simulink model "euler321_I2B_12B_with_contracts_ALL"  (R2019b)
settings: Solver=ode3  StartTime=0.0  StopTime=10.0  FixedStep=0.01  RelTol=1e-3  EnableMultiTasking=on
model workspace (MAT data in the model file):
  ContractValidatorBlocksMap : containers.Map (value not decoded)
undefined symbols (not defined in the file): contractAfterSimulation, contractBeforeSimulation, ContractBlock, ContractGuaranteeBlock, ContractValidatorBlock, saveValidatorParameters
libraries: cocosimLibs x1
(part 2 of 2)

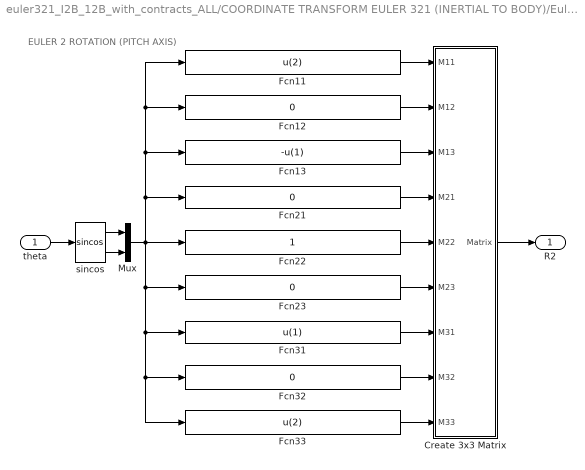
== system euler321_I2B_12B_with_contracts_ALL/COORDINATE TRANSFORM EULER 321 (INERTIAL TO BODY)/Euler 2 Rotation (Pitch) ==
  note: EULER 2 ROTATION (PITCH AXIS)
  theta : Inport
  Create 3x3 Matrix : Subsystem  mask(Create 3x3 Matrix){}
      mask help: shared_aeroblks:sharedaeroblkutil:blockCreate3x3MatrixDesc
      mask init:
      | if license('test','aerospace_blockset')
      |     aerosharedicon('shared');
      | elseif license('test','powertrain_blockset')
      |     sharedautoicon('shared');
      | end
      mask Help: eval('if license(''test'',''aerospace_blockset'')aerosharedhelp(''create_threebythree_matrix'');elseif license(''test'',''powertrain_blockset'')sharedautohelp(''create_threebythree_matrix'');end')
      mask Display:
      | port_label('input',1,'A_{11}','texmode','on');
      | port_label('input',2,'A_{12}','texmode','on');
      | port_label('input',3,'A_{13}','texmode','on');
      | port_label('input',4,'A_{21}','texmode','on');
      | port_label('input',5,'A_{22}','texmode','on');
      | port_label('input',6,'A_{23}','texmode','on');
      | port_label('input',7,'A_{31}','texmode','on');
      | port_label('input',8,'A_{32}','texmode','on');
      | port_label('input',9,'A_{33}','texmode','on');
      | port_label('output',1,'A','texmode','on');
  Fcn11 : Fcn  Expr=u(2)
  Fcn{12,21,23,32} (4 alike) : Fcn  Expr=0
  Fcn13 : Fcn  Expr=-u(1)
  Fcn22 : Fcn  Expr=1
  Fcn31 : Fcn  Expr=u(1)
  Fcn33 : Fcn  Expr=u(2)
  Mux : Mux  Inputs=2
  sincos : Trigonometry  Operator=sincos
  R2 : Outport  PortDimensions=[3,3]  VectorParamsAs1DForOutWhenUnconnected=off
  wires:
  theta/1 -> sincos/1
  Create 3x3 Matrix/1(Matrix) -> R2/1
  sincos/1 -> Mux/1
  sincos/2 -> Mux/2
  Mux/1 -> Fcn32/1, Fcn33/1, Fcn31/1, Fcn23/1, Fcn22/1, Fcn11/1, Fcn12/1, Fcn13/1, Fcn21/1
  Fcn11/1 -> Create 3x3 Matrix/1(M11)
  Fcn12/1 -> Create 3x3 Matrix/2(M12)
  Fcn13/1 -> Create 3x3 Matrix/3(M13)
  Fcn21/1 -> Create 3x3 Matrix/4(M21)
  Fcn31/1 -> Create 3x3 Matrix/7(M31)
  Fcn22/1 -> Create 3x3 Matrix/5(M22)
  Fcn23/1 -> Create 3x3 Matrix/6(M23)
  Fcn32/1 -> Create 3x3 Matrix/8(M32)
  Fcn33/1 -> Create 3x3 Matrix/9(M33)

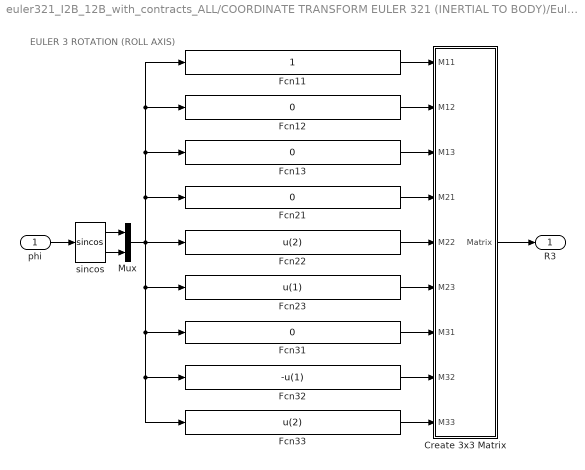
== system euler321_I2B_12B_with_contracts_ALL/COORDINATE TRANSFORM EULER 321 (INERTIAL TO BODY)/Euler 3 Rotation (Roll) ==
  note: EULER 3 ROTATION (ROLL AXIS)
  phi : Inport
  Create 3x3 Matrix : Subsystem  mask(Create 3x3 Matrix){}
      mask help: shared_aeroblks:sharedaeroblkutil:blockCreate3x3MatrixDesc
      mask init:
      | if license('test','aerospace_blockset')
      |     aerosharedicon('shared');
      | elseif license('test','powertrain_blockset')
      |     sharedautoicon('shared');
      | end
      mask Help: eval('if license(''test'',''aerospace_blockset'')aerosharedhelp(''create_threebythree_matrix'');elseif license(''test'',''powertrain_blockset'')sharedautohelp(''create_threebythree_matrix'');end')
      mask Display:
      | port_label('input',1,'A_{11}','texmode','on');
      | port_label('input',2,'A_{12}','texmode','on');
      | port_label('input',3,'A_{13}','texmode','on');
      | port_label('input',4,'A_{21}','texmode','on');
      | port_label('input',5,'A_{22}','texmode','on');
      | port_label('input',6,'A_{23}','texmode','on');
      | port_label('input',7,'A_{31}','texmode','on');
      | port_label('input',8,'A_{32}','texmode','on');
      | port_label('input',9,'A_{33}','texmode','on');
      | port_label('output',1,'A','texmode','on');
  Fcn11 : Fcn  Expr=1
  Fcn{12..13,21,31} (4 alike) : Fcn  Expr=0
  Fcn22 : Fcn  Expr=u(2)
  Fcn23 : Fcn  Expr=u(1)
  Fcn32 : Fcn  Expr=-u(1)
  Fcn33 : Fcn  Expr=u(2)
  Mux : Mux  Inputs=2
  sincos : Trigonometry  Operator=sincos
  R3 : Outport  PortDimensions=[3,3]  VectorParamsAs1DForOutWhenUnconnected=off
  wires:
  phi/1 -> sincos/1
  Create 3x3 Matrix/1(Matrix) -> R3/1
  sincos/1 -> Mux/1
  sincos/2 -> Mux/2
  Mux/1 -> Fcn32/1, Fcn33/1, Fcn31/1, Fcn23/1, Fcn22/1, Fcn11/1, Fcn12/1, Fcn13/1, Fcn21/1
  Fcn11/1 -> Create 3x3 Matrix/1(M11)
  Fcn12/1 -> Create 3x3 Matrix/2(M12)
  Fcn13/1 -> Create 3x3 Matrix/3(M13)
  Fcn21/1 -> Create 3x3 Matrix/4(M21)
  Fcn31/1 -> Create 3x3 Matrix/7(M31)
  Fcn22/1 -> Create 3x3 Matrix/5(M22)
  Fcn23/1 -> Create 3x3 Matrix/6(M23)
  Fcn32/1 -> Create 3x3 Matrix/8(M32)
  Fcn33/1 -> Create 3x3 Matrix/9(M33)

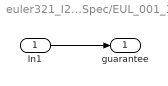
== system euler321_I2B_12B_with_contracts_ALL/euler321_I2B_12B_euler321_Spec/EUL_001_1 ==
  In1 : Inport
  guarantee : Outport  OutDataTypeStr=boolean
  wires:
  In1/1 -> guarantee/1

== system euler321_I2B_12B_with_contracts_ALL/euler321_I2B_12B_euler321_Spec/EUL_001_2 ==
  In1 : Inport
  guarantee : Outport  OutDataTypeStr=boolean
  wires:
  In1/1 -> guarantee/1

== system euler321_I2B_12B_with_contracts_ALL/euler321_I2B_12B_euler321_Spec/EUL_001_3 ==
  In1 : Inport
  guarantee : Outport  OutDataTypeStr=boolean
  wires:
  In1/1 -> guarantee/1

== system euler321_I2B_12B_with_contracts_ALL/euler321_I2B_12B_euler321_Spec/EUL_001_4 ==
  In1 : Inport
  guarantee : Outport  OutDataTypeStr=boolean
  wires:
  In1/1 -> guarantee/1

== system euler321_I2B_12B_with_contracts_ALL/euler321_I2B_12B_euler321_Spec/EUL_001_5 ==
  In1 : Inport
  guarantee : Outport  OutDataTypeStr=boolean
  wires:
  In1/1 -> guarantee/1

== system euler321_I2B_12B_with_contracts_ALL/euler321_I2B_12B_euler321_Spec/EUL_001_6 ==
  In1 : Inport
  guarantee : Outport  OutDataTypeStr=boolean
  wires:
  In1/1 -> guarantee/1

== system euler321_I2B_12B_with_contracts_ALL/euler321_I2B_12B_euler321_Spec/EUL_001_7 ==
  In1 : Inport
  guarantee : Outport  OutDataTypeStr=boolean
  wires:
  In1/1 -> guarantee/1

== system euler321_I2B_12B_with_contracts_ALL/euler321_I2B_12B_euler321_Spec/EUL_001_8 ==
  In1 : Inport
  guarantee : Outport  OutDataTypeStr=boolean
  wires:
  In1/1 -> guarantee/1

== system euler321_I2B_12B_with_contracts_ALL/euler321_I2B_12B_euler321_Spec/EUL_001_9 ==
  In1 : Inport
  guarantee : Outport  OutDataTypeStr=boolean
  wires:
  In1/1 -> guarantee/1

== system euler321_I2B_12B_with_contracts_ALL/euler321_I2B_12B_euler321_Spec/EUL_002_1 ==
  In1 : Inport
  guarantee : Outport  OutDataTypeStr=boolean
  wires:
  In1/1 -> guarantee/1

== system euler321_I2B_12B_with_contracts_ALL/euler321_I2B_12B_euler321_Spec/EUL_002_2 ==
  In1 : Inport
  guarantee : Outport  OutDataTypeStr=boolean
  wires:
  In1/1 -> guarantee/1

== system euler321_I2B_12B_with_contracts_ALL/euler321_I2B_12B_euler321_Spec/EUL_002_3 ==
  In1 : Inport
  guarantee : Outport  OutDataTypeStr=boolean
  wires:
  In1/1 -> guarantee/1

== system euler321_I2B_12B_with_contracts_ALL/euler321_I2B_12B_euler321_Spec/EUL_003 ==
  In1 : Inport
  guarantee : Outport  OutDataTypeStr=boolean
  wires:
  In1/1 -> guarantee/1

== system euler321_I2B_12B_with_contracts_ALL/euler321_I2B_12B_euler321_Spec/EUL_004 ==
  In1 : Inport
  guarantee : Outport  OutDataTypeStr=boolean
  wires:
  In1/1 -> guarantee/1

== system euler321_I2B_12B_with_contracts_ALL/euler321_I2B_12B_euler321_Spec/EUL_006_1 ==
  In1 : Inport
  guarantee : Outport  OutDataTypeStr=boolean
  wires:
  In1/1 -> guarantee/1

== system euler321_I2B_12B_with_contracts_ALL/euler321_I2B_12B_euler321_Spec/EUL_006_2 ==
  In1 : Inport
  guarantee : Outport  OutDataTypeStr=boolean
  wires:
  In1/1 -> guarantee/1

== system euler321_I2B_12B_with_contracts_ALL/euler321_I2B_12B_euler321_Spec/EUL_006_3 ==
  In1 : Inport
  guarantee : Outport  OutDataTypeStr=boolean
  wires:
  In1/1 -> guarantee/1

== system euler321_I2B_12B_with_contracts_ALL/euler321_I2B_12B_euler321_Spec/EUL_006_4 ==
  In1 : Inport
  guarantee : Outport  OutDataTypeStr=boolean
  wires:
  In1/1 -> guarantee/1

== system euler321_I2B_12B_with_contracts_ALL/euler321_I2B_12B_euler321_Spec/EUL_007 ==
  In1 : Inport
  guarantee : Outport  OutDataTypeStr=boolean
  wires:
  In1/1 -> guarantee/1

== system euler321_I2B_12B_with_contracts_ALL/euler321_I2B_12B_euler321_Spec/EUL_008 ==
  In1 : Inport
  guarantee : Outport  OutDataTypeStr=boolean
  wires:
  In1/1 -> guarantee/1

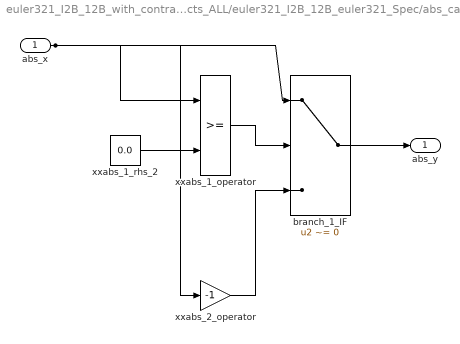
== system euler321_I2B_12B_with_contracts_ALL/euler321_I2B_12B_euler321_Spec/abs_call ==
  abs_x : Inport  OutDataTypeStr=double
  branch_1_IF : Switch  Criteria=u2 ~= 0
  xxabs_1_operator : RelationalOperator  OutDataTypeStr=boolean  RndMeth=Simplest
  xxabs_1_rhs_2 : Constant  Value=0.0  OutDataTypeStr=double
  xxabs_2_operator : Gain  Gain=-1  OutDataTypeStr=double
  abs_y : Outport
  wires:
  branch_1_IF/1 -> abs_y/1
  xxabs_1_rhs_2/1 -> xxabs_1_operator/2
  xxabs_2_operator/1 -> branch_1_IF/3
  xxabs_1_operator/1 -> branch_1_IF/2
  abs_x/1 -> xxabs_2_operator/1, xxabs_1_operator/1, branch_1_IF/1

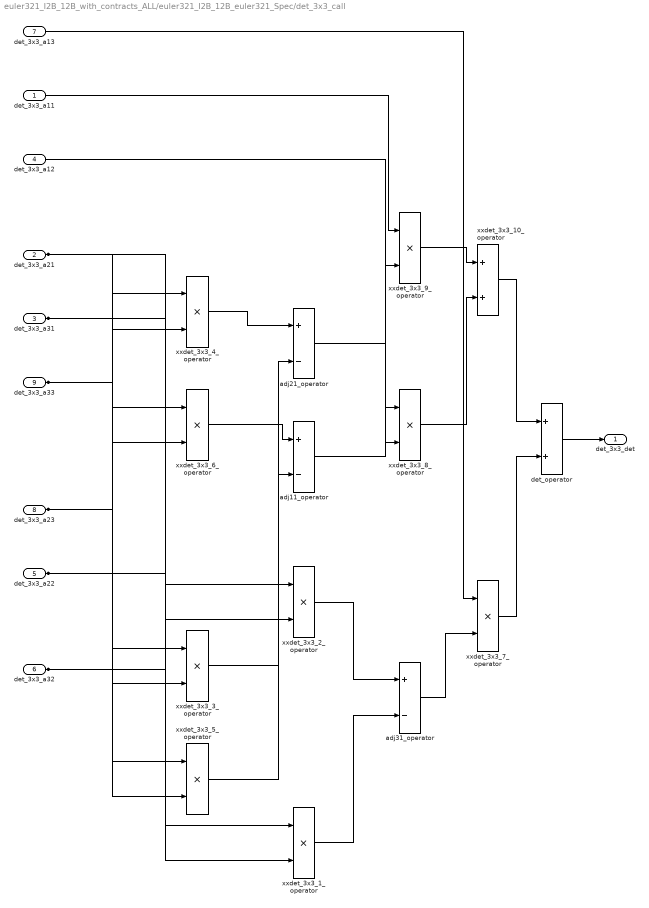
== system euler321_I2B_12B_with_contracts_ALL/euler321_I2B_12B_euler321_Spec/det_3x3_call ==
  det_3x3_a11 : Inport  OutDataTypeStr=double
  det_3x3_a21 : Inport  Port=2  OutDataTypeStr=double
  det_3x3_a31 : Inport  Port=3  OutDataTypeStr=double
  det_3x3_a12 : Inport  Port=4  OutDataTypeStr=double
  det_3x3_a22 : Inport  Port=5  OutDataTypeStr=double
  det_3x3_a32 : Inport  Port=6  OutDataTypeStr=double
  det_3x3_a13 : Inport  Port=7  OutDataTypeStr=double
  det_3x3_a23 : Inport  Port=8  OutDataTypeStr=double
  det_3x3_a33 : Inport  Port=9  OutDataTypeStr=double
  adj11_operator : Sum  Inputs=+-  OutDataTypeStr=double
  adj21_operator : Sum  Inputs=+-  OutDataTypeStr=double
  adj31_operator : Sum  Inputs=+-  OutDataTypeStr=double
  det_operator : Sum  OutDataTypeStr=double
  xxdet_3x3_10_operator : Sum  OutDataTypeStr=double
  xxdet_3x3_1_operator : Product  OutDataTypeStr=double
  xxdet_3x3_2_operator : Product  OutDataTypeStr=double
  xxdet_3x3_3_operator : Product  OutDataTypeStr=double
  xxdet_3x3_4_operator : Product  OutDataTypeStr=double
  xxdet_3x3_5_operator : Product  OutDataTypeStr=double
  xxdet_3x3_6_operator : Product  OutDataTypeStr=double
  xxdet_3x3_7_operator : Product  OutDataTypeStr=double
  xxdet_3x3_8_operator : Product  OutDataTypeStr=double
  xxdet_3x3_9_operator : Product  OutDataTypeStr=double
  det_3x3_det : Outport
  wires:
  det_operator/1 -> det_3x3_det/1
  adj11_operator/1 -> xxdet_3x3_9_operator/2
  det_3x3_a11/1 -> xxdet_3x3_9_operator/1
  adj21_operator/1 -> xxdet_3x3_8_operator/2
  det_3x3_a12/1 -> xxdet_3x3_8_operator/1
  adj31_operator/1 -> xxdet_3x3_7_operator/2
  det_3x3_a13/1 -> xxdet_3x3_7_operator/1
  xxdet_3x3_8_operator/1 -> xxdet_3x3_10_operator/2
  xxdet_3x3_9_operator/1 -> xxdet_3x3_10_operator/1
  xxdet_3x3_7_operator/1 -> det_operator/2
  xxdet_3x3_10_operator/1 -> det_operator/1
  xxdet_3x3_1_operator/1 -> adj31_operator/2
  xxdet_3x3_2_operator/1 -> adj31_operator/1
  xxdet_3x3_3_operator/1 -> adj21_operator/2
  xxdet_3x3_4_operator/1 -> adj21_operator/1
  xxdet_3x3_5_operator/1 -> adj11_operator/2
  xxdet_3x3_6_operator/1 -> adj11_operator/1
  det_3x3_a21/1 -> xxdet_3x3_3_operator/1, xxdet_3x3_2_operator/1
  det_3x3_a32/1 -> xxdet_3x3_5_operator/2, xxdet_3x3_2_operator/2
  det_3x3_a31/1 -> xxdet_3x3_4_operator/2, xxdet_3x3_1_operator/1
  det_3x3_a22/1 -> xxdet_3x3_6_operator/1, xxdet_3x3_1_operator/2
  det_3x3_a23/1 -> xxdet_3x3_5_operator/1, xxdet_3x3_4_operator/1
  det_3x3_a33/1 -> xxdet_3x3_6_operator/2, xxdet_3x3_3_operator/2

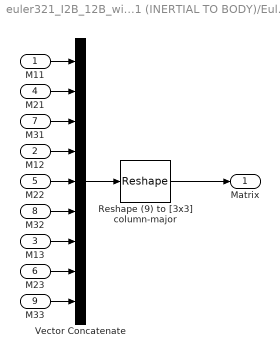
== system euler321_I2B_12B_with_contracts_ALL/COORDINATE TRANSFORM EULER 321 (INERTIAL TO BODY)/Euler 1 Rotation (Yaw)/Create 3x3 Matrix ==
  M11 : Inport  PortDimensions=1
  M12 : Inport  Port=2  PortDimensions=1
  M13 : Inport  Port=3  PortDimensions=1
  M21 : Inport  Port=4  PortDimensions=1
  M22 : Inport  Port=5  PortDimensions=1
  M23 : Inport  Port=6  PortDimensions=1
  M31 : Inport  Port=7  PortDimensions=1
  M32 : Inport  Port=8  PortDimensions=1
  M33 : Inport  Port=9  PortDimensions=1
  Reshape (9) to [3x3] column-major : Reshape  OutputDimensionality=Customize  OutputDimensions=[3,3]
  Vector Concatenate : Concatenate  NumInputs=9
  Matrix : Outport  PortDimensions=[3 3]  VectorParamsAs1DForOutWhenUnconnected=off
  wires:
  M33/1 -> Vector Concatenate/9
  M23/1 -> Vector Concatenate/8
  M13/1 -> Vector Concatenate/7
  M32/1 -> Vector Concatenate/6
  Reshape (9) to [3x3] column-major/1 -> Matrix/1
  M22/1 -> Vector Concatenate/5
  M12/1 -> Vector Concatenate/4
  M31/1 -> Vector Concatenate/3
  M21/1 -> Vector Concatenate/2
  M11/1 -> Vector Concatenate/1
  Vector Concatenate/1 -> Reshape (9) to [3x3] column-major/1

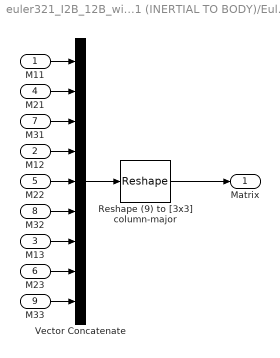
== system euler321_I2B_12B_with_contracts_ALL/COORDINATE TRANSFORM EULER 321 (INERTIAL TO BODY)/Euler 2 Rotation (Pitch)/Create 3x3 Matrix ==
  M11 : Inport  PortDimensions=1
  M12 : Inport  Port=2  PortDimensions=1
  M13 : Inport  Port=3  PortDimensions=1
  M21 : Inport  Port=4  PortDimensions=1
  M22 : Inport  Port=5  PortDimensions=1
  M23 : Inport  Port=6  PortDimensions=1
  M31 : Inport  Port=7  PortDimensions=1
  M32 : Inport  Port=8  PortDimensions=1
  M33 : Inport  Port=9  PortDimensions=1
  Reshape (9) to [3x3] column-major : Reshape  OutputDimensionality=Customize  OutputDimensions=[3,3]
  Vector Concatenate : Concatenate  NumInputs=9
  Matrix : Outport  PortDimensions=[3 3]  VectorParamsAs1DForOutWhenUnconnected=off
  wires:
  M33/1 -> Vector Concatenate/9
  M23/1 -> Vector Concatenate/8
  M13/1 -> Vector Concatenate/7
  M32/1 -> Vector Concatenate/6
  Reshape (9) to [3x3] column-major/1 -> Matrix/1
  M22/1 -> Vector Concatenate/5
  M12/1 -> Vector Concatenate/4
  M31/1 -> Vector Concatenate/3
  M21/1 -> Vector Concatenate/2
  M11/1 -> Vector Concatenate/1
  Vector Concatenate/1 -> Reshape (9) to [3x3] column-major/1

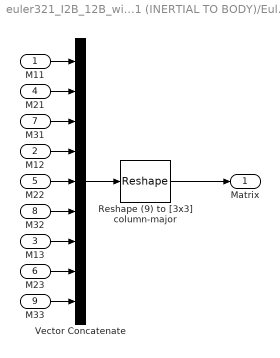
== system euler321_I2B_12B_with_contracts_ALL/COORDINATE TRANSFORM EULER 321 (INERTIAL TO BODY)/Euler 3 Rotation (Roll)/Create 3x3 Matrix ==
  M11 : Inport  PortDimensions=1
  M12 : Inport  Port=2  PortDimensions=1
  M13 : Inport  Port=3  PortDimensions=1
  M21 : Inport  Port=4  PortDimensions=1
  M22 : Inport  Port=5  PortDimensions=1
  M23 : Inport  Port=6  PortDimensions=1
  M31 : Inport  Port=7  PortDimensions=1
  M32 : Inport  Port=8  PortDimensions=1
  M33 : Inport  Port=9  PortDimensions=1
  Reshape (9) to [3x3] column-major : Reshape  OutputDimensionality=Customize  OutputDimensions=[3,3]
  Vector Concatenate : Concatenate  NumInputs=9
  Matrix : Outport  PortDimensions=[3 3]  VectorParamsAs1DForOutWhenUnconnected=off
  wires:
  M33/1 -> Vector Concatenate/9
  M23/1 -> Vector Concatenate/8
  M13/1 -> Vector Concatenate/7
  M32/1 -> Vector Concatenate/6
  Reshape (9) to [3x3] column-major/1 -> Matrix/1
  M22/1 -> Vector Concatenate/5
  M12/1 -> Vector Concatenate/4
  M31/1 -> Vector Concatenate/3
  M21/1 -> Vector Concatenate/2
  M11/1 -> Vector Concatenate/1
  Vector Concatenate/1 -> Reshape (9) to [3x3] column-major/1
